simulink model "Truth_Table"  (R2025b)
settings: Solver=FixedStepDiscrete  StartTime=0.0  StopTime=10.0  FixedStep=0.01  RelTol=1e-3
libraries: simulink x1
settings Model: Creator=soura  LastModifiedBy=soura

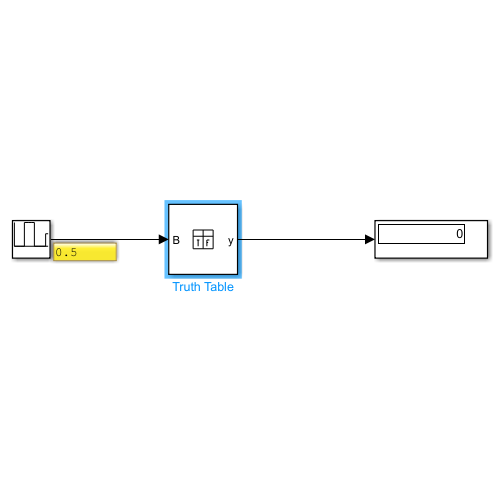
[thumbnail: Simulink's stored preview of the top-level diagram]
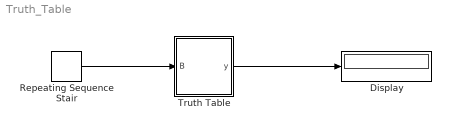
== system Truth_Table ==
  Display : Display
  Repeating Sequence Stair : simulink/Sources/Repeating Sequence Stair  OutValues=[0 0 0 1 1 1 0 0 0 0.5].'  tsamp=-1  OutMin=[]  OutMax=[]  OutDataTypeStr=double  OutputDataTypeScalingMode=double  OutDataType=fixdt(0,8)  ConRadixGroup=Best Precision: Vector-wise  OutScaling=2^-12
  Truth Table : Truth Table  TreatAsAtomicUnit=on
  wires:
  Repeating Sequence Stair/1 -> Truth Table/1(B)
  Truth Table/1(y) -> Display/1

== matlab function Truth_Table/Truth Table ==
  data: B input; y output
function y = fcn(B)

aVarTruthTableCondition_1 = false;
aVarTruthTableCondition_2 = false;


% Example condition 1

aVarTruthTableCondition_1 = logical(B==1);

% Example condition 2

aVarTruthTableCondition_2 = logical(B==0);

if (~aVarTruthTableCondition_1 && aVarTruthTableCondition_2)
    aFcnTruthTableAction_1();
elseif (aVarTruthTableCondition_1 && ~aVarTruthTableCondition_2)
    aFcnTruthTableAction_2();
else % Default
    aFcnTruthTableAction_1();
end

function aFcnTruthTableAction_1()

    % Example action 1 called from D1 & D2 column in condition table

    y = 0;

function aFcnTruthTableAction_2()

    % Example action 2 called from D3 column in condition table

    y = 1;
